simulink model "deadlock_ROS"  (R2025b)
settings: Solver=FixedStepAuto  StartTime=0.0  StopTime=30  RelTol=1e-3
libraries: robotlib x6
settings Model: Creator=nirmay  LastModifiedBy=simongou
settings OptimizationCC: DefaultParameterBehavior=Inlined  EnhancedBackFolding=on  PassReuseOutputArgsAs=Individual arguments  ZeroExternalMemoryAtStartup=off  ZeroInternalMemoryAtStartup=off  MaxStackSize=64  OptimizeBlockOrder=speed  DifferentSizesBufferReuse=on  OptimizationCustomize=off  EfficientTunableParamExpr=on
settings DebuggingCC: ParameterTunabilityLossMsg=error
settings HardwareCC: ProdBitPerPointer=32.0  ProdBitPerSizeT=32.0  ProdBitPerPtrDiffT=32.0  ProdLargestAtomicFloat=None  ProdIntDivRoundTo=Undefined  ProdEndianess=Unspecified  ProdWordSize=32.0  ProdHWDeviceType=Generic->Unspecified (assume 32-bit Generic)
settings SFSimCC: MATLABDynamicMemAlloc=off
settings RTWCC: SystemTargetFile=ert.tlc  HardwareBoard=Robot Operating System (ROS)  TLCOptions="-aInlineSetEventsForThisBaseRateFcn=TLC_FALSE -aSuppressMultiTaskScheduler=TLC_FALSE  -aRateBasedStepFcn=0"  TemplateMakefile=ert_default_tmf  Toolchain=Catkin  TargetLang=C++  Description=Embedded Coder
settings CodeAppCC: ForceParamTrailComments=on  IgnoreCustomStorageClasses=off  OperatorAnnotations=on  SimulinkDataObjDesc=on  SFDataObjDesc=on  InsertBlockDesc=on

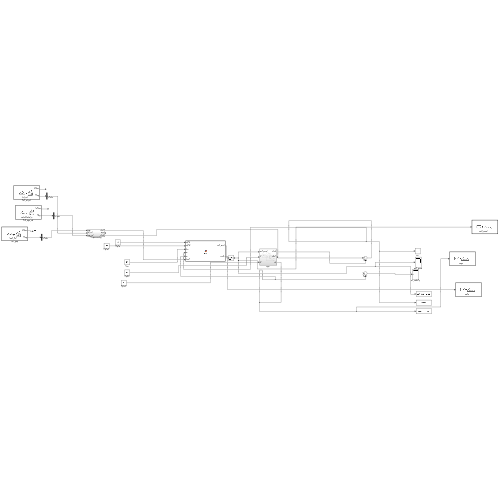
[thumbnail: Simulink's stored preview of the top-level diagram]
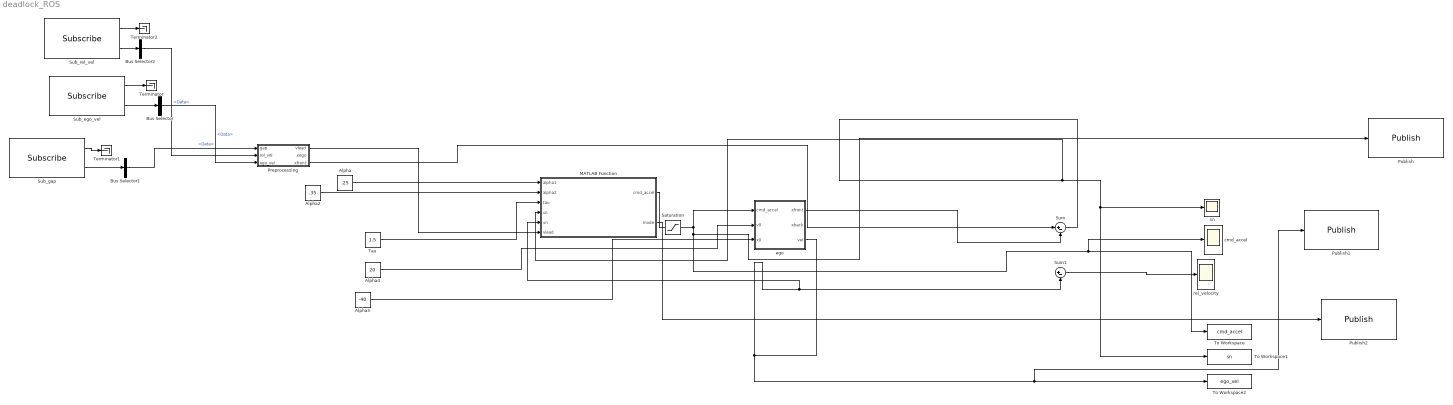
== system deadlock_ROS ==
  Alpha : Constant  Value=.25
  Alpha2 : Constant  Value=.35
  Alpha4 : Constant  Value=20
  Alpha5 : Constant  Value=-40
  Bus Selector : BusSelector  OutputSignals=Data
  Bus Selector1 : BusSelector  OutputSignals=Data
  Bus Selector2 : BusSelector  OutputSignals=Data
  MATLAB Function : MATLAB Function  TreatAsAtomicUnit=on
  Preprocessing : Subsystem
  Publish : robotlib/Publish  topicSource=Specify your own  topic=cmd_accel  messageType=std_msgs/Float64  legacyBusStruct=off  messageQueueLength=1
  Publish1 : robotlib/Publish  topicSource=Specify your own  topic=vego  messageType=std_msgs/Float64  legacyBusStruct=off  messageQueueLength=1
  Publish2 : robotlib/Publish  topicSource=Specify your own  topic=mode  messageType=std_msgs/Int32  legacyBusStruct=off  messageQueueLength=1
  Saturation : Saturate  UpperLimit=1.5  LowerLimit=-3.0
  Sub_ego_vel : robotlib/Subscribe  topicSource=Specify your own  topic=car/state/vel_x  messageType=std_msgs/Float64  SampleTime=-1  legacyBusStruct=off  messageQueueLength=1
  Sub_gap : robotlib/Subscribe  topicSource=Specify your own  topic=lead_dist  messageType=std_msgs/Float64  SampleTime=-1  legacyBusStruct=off  messageQueueLength=1
  Sub_rel_vel : robotlib/Subscribe  topicSource=Specify your own  topic=/rel_vel  messageType=std_msgs/Float64  SampleTime=-1  legacyBusStruct=off  messageQueueLength=1
  Sum : Sum  Inputs=|+-
  Sum1 : Sum  Inputs=|+-
  Tau : Constant  Value=1.5
  Terminator : Terminator
  Terminator1 : Terminator
  Terminator2 : Terminator
  To Workspace : ToWorkspace  VariableName=cmd_accel  SaveFormat=Timeseries  SampleTime=-1
  To Workspace1 : ToWorkspace  VariableName=sn  SaveFormat=Timeseries  SampleTime=-1
  To Workspace2 : ToWorkspace  VariableName=ego_vel  SaveFormat=Timeseries  SampleTime=-1
  cmd_accel : Scope
      settings: ActiveDisplayYMinimum=-0.80741599020341992  ActiveDisplayYMaximum=2.3119351100226022  DataLoggingVariableName=ScopeData2
  ego : Subsystem
  rel_velocity : Scope
      settings: ActiveDisplayYMinimum=-0.63030265545268038  ActiveDisplayYMaximum=5.6255891839391863
  sn : Scope
      settings: ActiveDisplayYMinimum=-2.4871584438129148  ActiveDisplayYMaximum=22.48009769464
  wires:
  ego/1(xfront) -> Sum/2
  MATLAB Function/1(cmd_accel) -> To Workspace/1, cmd_accel/1, Publish/1, ego/1(cmd_accel)
  Sum/1 -> MATLAB Function/4(sn), To Workspace1/1, sn/1
  Alpha/1 -> MATLAB Function/1(alpha1)
  Tau/1 -> MATLAB Function/3(tau)
  Alpha4/1 -> ego/2(v0)
  Alpha5/1 -> ego/3(x0)
  ego/3(vel) -> Sum1/2, MATLAB Function/5(vn), Publish1/1, To Workspace2/1
  Alpha2/1 -> MATLAB Function/2(alpha2)
  Sum1/1 -> rel_velocity/1
  Bus Selector2/1 -> Preprocessing/2(rel_vel)  "<Data>"
  Sub_rel_vel/2 -> Bus Selector2/1
  Bus Selector/1 -> Preprocessing/3(ego_vel)  "<Data>"
  Sub_gap/1 -> Terminator1/1
  Bus Selector1/1 -> Preprocessing/1(gap)  "<Data>"
  Sub_gap/2 -> Bus Selector1/1
  Sub_ego_vel/1 -> Terminator/1
  Sub_ego_vel/2 -> Bus Selector/1
  Preprocessing/3(xfront) -> Sum/1
  Preprocessing/1(vlead) -> MATLAB Function/6(vlead)
  Sub_rel_vel/1 -> Terminator2/1
  MATLAB Function/2(mode) -> Publish2/1

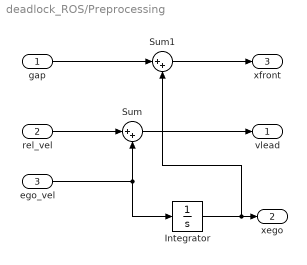
== system deadlock_ROS/Preprocessing ==
  gap : Inport
  rel_vel : Inport  Port=2
  ego_vel : Inport  Port=3
  Integrator : Integrator
  Sum : Sum  Inputs=|++
  Sum1 : Sum  Inputs=|++
  vlead : Outport
  xego : Outport  Port=2
  xfront : Outport  Port=3
  wires:
  rel_vel/1 -> Sum/1
  Sum/1 -> vlead/1
  Integrator/1 -> Sum1/2, xego/1
  ego_vel/1 -> Integrator/1, Sum/2
  gap/1 -> Sum1/1
  Sum1/1 -> xfront/1

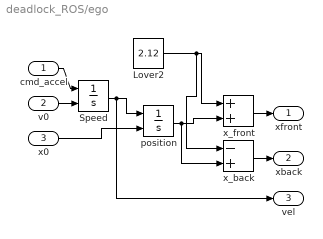
== system deadlock_ROS/ego ==
  cmd_accel : Inport
  v0 : Inport  Port=2
  x0 : Inport  Port=3
  Lover2 : Constant  Value=2.12
  Speed : Integrator  InitialConditionSource=external
  position : Integrator  InitialConditionSource=external
  x_back : Sum  Inputs=-+
  x_front : Sum
  xfront : Outport
  xback : Outport  Port=2
  vel : Outport  Port=3
  wires:
  x_front/1 -> xfront/1
  x_back/1 -> xback/1
  v0/1 -> Speed/2
  x0/1 -> position/2
  cmd_accel/1 -> Speed/1
  position/1 -> x_back/2, x_front/2
  Speed/1 -> vel/1, position/1
  Lover2/1 -> x_back/1, x_front/1

== matlab function deadlock_ROS/MATLAB Function ==
  data: alpha1 input; alpha2 input; tau input; cmd_accel output; sn input; vn input; vlead input; mode output
function [cmd_accel, mode] = fcn(alpha1, alpha2, tau, sn, vn, vlead)
wfunction [cmd_accel, mode] = fcn(alpha1, alpha2, tau, sn, vn, vlead)

% Mode 1=NORMAL, 2=CLOSING, 3=GROWING, 4=EMERGENCY, 5=STOP_HOLD


s0        = 5.0;     % standstill distance (m)
B_emg     = 5.0;     % max braking allowed 
amin_norm = -3.0;    % normal braking limit
amax      =  2.0;    % acceleration limit
ttc_min   = 1.2;     % Time to Collision threshold for emergency (s)
v_stop    = 0.2;     % near-stop (m/s)
s_hold    = s0 + 0.5;

if vlead <= 0
    vlead = vn;   % treat as same speed; disables closing trigger
end


if any(isnan([sn vn vlead])) || any(isinf([sn vn vlead]))
    cmd_accel = 0; mode = 1; return;
end
vn      = max(vn,0);               % never let negative ego speed skew math
rel_vel = vlead - vn;              

% Safe distance includes: standstill + time-gap + stopping distance
s_ref_hw   = s0 + tau * vn;                  % headway term
s_brake    = (vn^2) / (2 * B_emg);           % distance needed to stop
s_safe     = s_ref_hw + s_brake;             % start braking before it's too late

% normal situation
if (sn < s_ref_hw && rel_vel < 0)
    mode = 2;  a1 = alpha1*1.0; a2 = alpha2*1.8;
elseif (sn > 1.5*s_ref_hw && rel_vel > 0)
    mode = 3;  a1 = alpha1*0.8; a2 = alpha2*0.6;
else
    mode = 1;  a1 = alpha1;     a2 = alpha2;
end
u_base = a1*(sn - s_ref_hw) + a2*rel_vel;

% predictive braking if getting close to a crash
is_closing = (rel_vel < 0);
if is_closing && sn > 0
    ttc = sn / (-rel_vel);
else
    ttc = inf;
end

emergency = (sn <= s0) ...                 % too close, might crash
         || (sn < s_brake + s0) ...        % Need to brake now to avoid crash
         || (isfinite(ttc) && ttc < ttc_min);

if emergency
    mode = 4;
    % Allow emergency braking if needed
    u_eb = -B_emg;
    cmd_accel = max(u_eb, u_base);
else
    % If not an emergency situation, don't max deceleration
    cmd_accel = min(max(u_base, amin_norm), amax);
end

% Don't allow negative velocity when car in front is stopped
if (vn < v_stop) && (sn < s_hold) && (rel_vel >= 0)
    mode = 5;
    cmd_accel = 0;
end

% safety to avoid excessive dedcel
cmd_accel = min(max(cmd_accel, -B_emg), amax);

%reduce variability in cmd_accel
if abs(cmd_accel) < 0.05
    cmd_accel = 0;
end
end
